simulink subsystem "ConventionalVehicleSSC"  (R2023b)
settings: Solver=VariableStepAuto  StartTime=0.0  StopTime=10.0  RelTol=1e-3
libraries: fl_lib x3, nesl_utility_internal x1
settings Model: Creator=The MathWorks, Inc.  LastModifiedBy=The MathWorks, Inc.

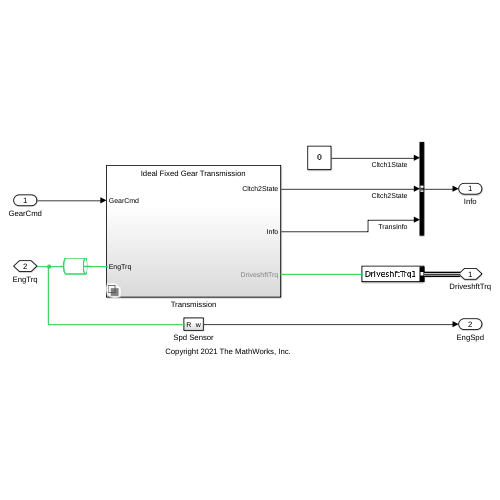
[thumbnail: Simulink's stored preview of the top-level diagram]
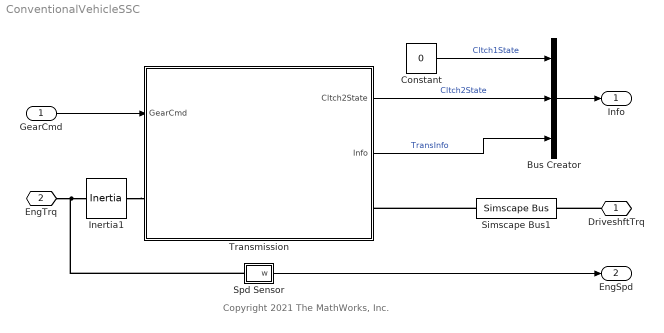
== system ConventionalVehicleSSC ==
  note: Copyright 2021 The MathWorks, Inc.
  GearCmd : Inport
  Bus Creator : BusCreator  Inputs=3
  Constant : Constant  Value=0  SampleTime=-1
  Inertia1 : fl_lib/Mechanical/Rotational Elements/Inertia  inertia=PlntEngInertia kg*m^2  num_ports=foundation.enum.numPorts2.two  w_specify=off  w_priority=High  w=0 rad/s  w_nominal_specify=off  w_nominal_unit=rad/s  w_nominal_value=1  t_specify=off  t_priority=None  t=0 N*m  t_nominal_specify=off  t_nominal_unit=N*m  t_nominal_value=1
      settings: InternalSimscapePortConfiguration="{\"Bottom\":[],\"Left\":[{\"id\":\"I\",\"label\":\"\",\"type\":\"foundation.mechanical.rotational.rotational\"}],\"Right\":[{\"id\":\"J\",\"label\":\"\",\"type\":\"foundation.mechanical.rotational.rotational\"}],\"Top\":[]}"
  Simscape Bus1 : SimscapeBus  HierarchyStrings=DriveshftTrq1
  Spd Sensor : Subsystem
  Transmission : Subsystem  Variant=on  VariantControlMode=label  VariantControl=1  LabelModeActiveChoice=Ideal Fixed Gear Transmission
  DriveshftTrq : PMIOPort  Side=Right
  EngTrq : PMIOPort  Port=2  Side=Left
  Info : Outport
  EngSpd : Outport  Port=2
  wires:
  Spd Sensor/1(w) -> EngSpd/1
  Bus Creator/1 -> Info/1
  GearCmd/1 -> Transmission/1(GearCmd)
  Transmission/1(Cltch2State) -> Bus Creator/2  "Cltch2State"
  Transmission/2(Info) -> Bus Creator/3  "TransInfo"
  Constant/1 -> Bus Creator/1  "Cltch1State"
  connections:
  Inertia1/RConn1 -- Spd Sensor/LConn1 -- EngTrq/RConn1
  Simscape Bus1/LConn1 -- Transmission/RConn1
  Inertia1/LConn1 -- Transmission/LConn1
  DriveshftTrq/RConn1 -- Simscape Bus1/RConn1

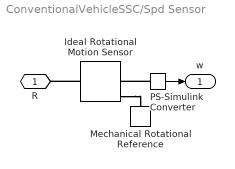
== system ConventionalVehicleSSC/Spd Sensor ==
  Ideal Rotational Motion Sensor : fl_lib/Mechanical/Mechanical Sensors/Ideal Rotational Motion Sensor  reference=foundation.enum.MeasurementReference.difference  acceleration_port=false  velocity_port=true  position_port=true  wrap_angle=simscape.enum.onoff.off  offset=0 rad
  Mechanical Rotational Reference : fl_lib/Mechanical/Rotational Elements/Mechanical Rotational Reference
  PS-Simulink Converter : nesl_utility_internal/PS-Simulink Converter  PhysicalDomain=network_engine_domain  SubClassName=ps_output  LeftPortType=input  RightPortType=output  PseudoPeriodic=off  Frequencies=[]  VectorFormat=inherit  Unit=inherit  AffineConversion=off
  R : PMIOPort  Side=Left
  w : Outport
  wires:
  PS-Simulink Converter/1 -> w/1
  connections:
  PS-Simulink Converter/LConn1 -- Ideal Rotational Motion Sensor/RConn2
  Ideal Rotational Motion Sensor/LConn1 -- R/RConn1
  Ideal Rotational Motion Sensor/RConn1 -- Mechanical Rotational Reference/LConn1

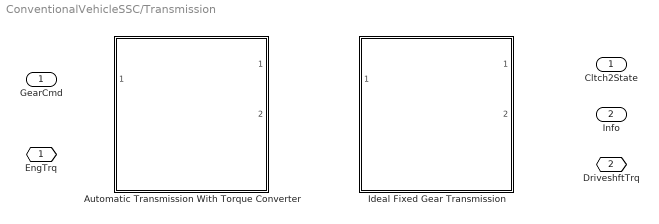
== system ConventionalVehicleSSC/Transmission ==
  GearCmd : Inport
  Automatic Transmission With Torque Converter : Subsystem  VariantControl=Automatic Transmission With Torque Converter  ReferencedSubsystem=AutomaticTransmissionWithTorqueConverterSSC
  Ideal Fixed Gear Transmission : Subsystem  VariantControl=Ideal Fixed Gear Transmission  ReferencedSubsystem=IdealFixedGearTransmissionSSC
  EngTrq : PMIOPort  Side=Left
  DriveshftTrq : PMIOPort  Port=2  Side=Right
  Cltch2State : Outport
  Info : Outport  Port=2
